simulink model "Magnetorquers"  (R2023b)
settings: Solver=FixedStepAuto  StartTime=0.0  StopTime=10.0  FixedStep=0.001  RelTol=1e-3
model workspace (MAT data in the model file):
  M1_Gain = 8.4
  M1_I_max = 0.075
  M1_V = 5
  M2_Gain = 8.4
  M2_I_max = 0.075
  M2_V = 5
settings Model: Creator=andrea  LastModifiedBy=andrea

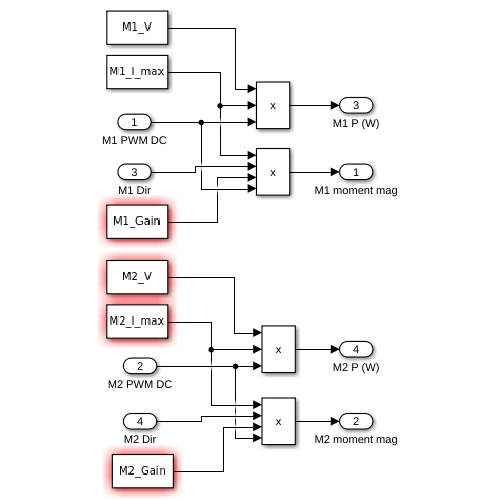
[thumbnail: Simulink's stored preview of the top-level diagram]
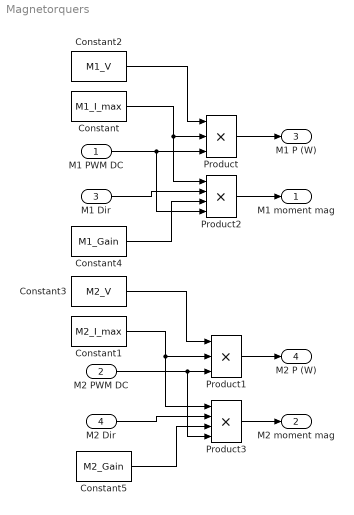
== system Magnetorquers ==
  M1 PWM DC : Inport
  M2 PWM DC : Inport  Port=2
  M1 Dir : Inport  Port=3
  M2 Dir : Inport  Port=4
  Constant : Constant  Value=M1_I_max
  Constant1 : Constant  Value=M2_I_max
  Constant2 : Constant  Value=M1_V
  Constant3 : Constant  Value=M2_V
  Constant4 : Constant  Value=M1_Gain
  Constant5 : Constant  Value=M2_Gain
  Product : Product  Inputs=3
  Product1 : Product  Inputs=3
  Product2 : Product  Inputs=4
  Product3 : Product  Inputs=4
  M1 moment mag : Outport
  M2 moment mag : Outport  Port=2
  M1 P (W) : Outport  Port=3
  M2 P (W) : Outport  Port=4
  wires:
  Constant5/1 -> Product3/3
  M1 Dir/1 -> Product2/2
  M2 Dir/1 -> Product3/2
  Product1/1 -> M2 P (W)/1
  M2 PWM DC/1 -> Product3/4, Product1/3
  Product3/1 -> M2 moment mag/1
  Product2/1 -> M1 moment mag/1
  Constant3/1 -> Product1/1
  Constant/1 -> Product2/1, Product/2
  M1 PWM DC/1 -> Product2/4, Product/3
  Constant2/1 -> Product/1
  Constant1/1 -> Product3/1, Product1/2
  Constant4/1 -> Product2/3
  Product/1 -> M1 P (W)/1
